simulink model "nms_model"  (Simulink 7.5)
settings: Solver=ode15s  StartTime=0.0  StopTime=60  FixedStep=1e-3  MaxStep=ts_max  RelTol=1e-3  AbsTol=1e-4
InitFcn:
  | nms_model_MechInit
  | nms_model_ControlInit
values from neighbouring files (symbols this model uses):
  c = 0.05    [muscleParams.m]    (also in nms_model_MechInit.m)
  c_jointstop = 0.3 / (pi/180)    (= 17.1887338539)    [muscleParams.m]    (also in nms_model_MechInit.m)
  D12_F = 0.16    [nms_model_MechInit.m]
  D12_S = L_S    (= 0.5)    [nms_model_MechInit.m]
  D12_T = L_T    (= 0.5)    [nms_model_MechInit.m]
  D13_F = 0.20    (= 0.2)    [nms_model_MechInit.m]
  D1G_F = 0.14    [nms_model_MechInit.m]
  D1G_HAT = 0.35    [nms_model_MechInit.m]
  D1G_S = 0.3    [nms_model_MechInit.m]
  D1G_T = 0.3    [nms_model_MechInit.m]
  DeltaThRef = 5e-3    (= 0.005)    [nms_model_MechInit.m]
  eref = 0.04    [muscleParams.m]    (also in nms_model_MechInit.m)
  FmaxGAS = 1500    [nms_model_MechInit.m]
  FmaxGLU = 1500    [nms_model_MechInit.m]
  FmaxHAM = 3000    [nms_model_MechInit.m]
  FmaxHFL = 2000    [nms_model_MechInit.m]
  FmaxSOL = 4000    [nms_model_MechInit.m]
  FmaxTA = 800    [nms_model_MechInit.m]
  FmaxVAS = 300    [muscleParams.m]    (also in nms_model_MechInit.m = 6000)
  GainDeltaTheta = 2 /100*180/pi    (= 1.14591559026)    [nms_model_ControlInit.m]
  GainGAS = 1.1/FmaxGAS    [nms_model_ControlInit.m]
  GainGLU = 0.5/FmaxGLU    [nms_model_ControlInit.m]
  GainHAM = 0.65/FmaxHAM    [nms_model_ControlInit.m]
  GainHAMHFL = 4    [nms_model_ControlInit.m]
  GainHFL = 0.5    [nms_model_ControlInit.m]
  GainKneOverExt = 2    [nms_model_ControlInit.m]
  GainSOL = 1.2/FmaxSOL    [nms_model_ControlInit.m]
  GainSOLTA = 0.4/FmaxSOL    [nms_model_ControlInit.m]
  GainTA = 1.1    [nms_model_ControlInit.m]
  GainVAS = 1.2/FmaxVAS    [nms_model_ControlInit.m]
  In_F = 0.005    [nms_model_MechInit.m]
  In_HAT = 3    [nms_model_MechInit.m]
  In_S = 0.05    [nms_model_MechInit.m]
  In_T = 0.15    [nms_model_MechInit.m]
  K = 5    [muscleParams.m]    (also in nms_model_MechInit.m)
  k_gx = (2*(m_F+m_S+m_T)+m_HAT)*g/0.1    (= 7848)    [nms_model_MechInit.m]
  k_gy = (2*(m_F+m_S+m_T)+m_HAT)*g/0.01    (= 78480)    [nms_model_MechInit.m]
  k_pressure = m_HAT * 9.81 / DeltaThRef    (= 104967)    [nms_model_MechInit.m]
  K_swing = 0.25    [nms_model_ControlInit.m]
  KneePh23Offset = 170*pi/180    (= 2.96705972839)    [nms_model_ControlInit.m]
  LceOffsetHAM = 0.85    [nms_model_ControlInit.m]
  LceOffsetHFL = 0.65    [nms_model_ControlInit.m]
  LceOffsetTA = 1-0.5*w    [nms_model_ControlInit.m]
  LongDelay = 0.020    (= 0.02)    [nms_model_ControlInit.m]
  loptGAS = 0.05    [nms_model_MechInit.m]
  loptGLU = 0.11    [nms_model_MechInit.m]
  loptHAM = 0.10    (= 0.1)    [nms_model_MechInit.m]
  loptHFL = 0.11    [nms_model_MechInit.m]
  loptSOL = 0.04    [nms_model_MechInit.m]
  loptTA = 0.06    [nms_model_MechInit.m]
  loptVAS = 0.13    [muscleParams.m]    (also in nms_model_MechInit.m = 0.08)
  lslackGAS = 0.40    (= 0.4)    [nms_model_MechInit.m]
  lslackGLU = 0.13    [nms_model_MechInit.m]
  lslackHAM = 0.31    [nms_model_MechInit.m]
  lslackHFL = 0.10    (= 0.1)    [nms_model_MechInit.m]
  lslackSOL = 0.26    [nms_model_MechInit.m]
  lslackTA = 0.24    [nms_model_MechInit.m]
  lslackVAS = 0.23    [muscleParams.m]    (also in nms_model_MechInit.m)
  m_F = 1.25    [nms_model_MechInit.m]
  m_HAT = 53.5    [nms_model_MechInit.m]
  m_S = 3.5    [nms_model_MechInit.m]
  m_T = 8.5    [nms_model_MechInit.m]
  MidDelay = 0.010    (= 0.01)    [nms_model_ControlInit.m]
  mu_slide = 0.8    [nms_model_MechInit.m]
  mu_stick = 0.9    [nms_model_MechInit.m]
  N = 1.5    [muscleParams.m]    (also in nms_model_MechInit.m)
  phi12_LowLimit = 70*pi/180    (= 1.2217304764)    [nms_model_MechInit.m]
  phi12_UpLimit = 180*pi/180    (= 3.14159265359)    [muscleParams.m]    (also in nms_model_MechInit.m = 2.26892802759)
  phi23_UpLimit = 159*pi/180    (= 2.77507351067)    [muscleParams.m]    (also in nms_model_MechInit.m = 3.05432619099)
  phi34_UpLimit = 230*pi/180    (= 4.01425727959)    [nms_model_MechInit.m]
  phimaxGASa = 110*pi/180    (= 1.91986217719)    [nms_model_MechInit.m]
  phimaxGASk = 140*pi/180    (= 2.44346095279)    [nms_model_MechInit.m]
  phimaxHAMk = 180*pi/180    (= 3.14159265359)    [nms_model_MechInit.m]
  phimaxSOL = 110*pi/180    (= 1.91986217719)    [nms_model_MechInit.m]
  phimaxTA = 80*pi/180    (= 1.3962634016)    [nms_model_MechInit.m]
  phimaxVAS = 90*pi/180    (= 1.57079632679)    [muscleParams.m]    (also in nms_model_MechInit.m = 2.87979326579)
  phirefGASa = 80*pi/180    (= 1.3962634016)    [nms_model_MechInit.m]
  phirefGASk = 165*pi/180    (= 2.87979326579)    [nms_model_MechInit.m]
  phirefGLU = 150*pi/180    (= 2.61799387799)    [nms_model_MechInit.m]
  phirefHAMh = 155*pi/180    (= 2.70526034059)    [nms_model_MechInit.m]
  phirefHAMk = 180*pi/180    (= 3.14159265359)    [nms_model_MechInit.m]
  phirefHFL = 180*pi/180    (= 3.14159265359)    [nms_model_MechInit.m]
  phirefSOL = 80*pi/180    (= 1.3962634016)    [nms_model_MechInit.m]
  phirefTA = 110*pi/180    (= 1.91986217719)    [nms_model_MechInit.m]
  phirefVAS = 60*pi/180    (= 1.0471975512)    [muscleParams.m]    (also in nms_model_MechInit.m = 2.18166156499)
  PosGainGG = 1/(30*pi/180)    (= 1.9098593171)    [nms_model_ControlInit.m]
  PreStimGAS = 0.01    [nms_model_ControlInit.m]
  PreStimGG = 0.05    [nms_model_ControlInit.m]
  PreStimGLU = 0.01    [nms_model_ControlInit.m]
  PreStimHAM = 0.01    [nms_model_ControlInit.m]
  PreStimHFL = 0.01    [nms_model_ControlInit.m]
  PreStimSOL = 0.01    [nms_model_ControlInit.m]
  PreStimTA = 0.01    [nms_model_ControlInit.m]
  PreStimVAS = 0.08    [nms_model_ControlInit.m]
  rGASa = 0.05    [nms_model_MechInit.m]
  rGASk = 0.05    [nms_model_MechInit.m]
  rGLU = 0.10    (= 0.1)    [nms_model_MechInit.m]
  rHAMh = 0.08    [nms_model_MechInit.m]
  rHAMk = 0.05    [nms_model_MechInit.m]
  rHFL = 0.10    (= 0.1)    [nms_model_MechInit.m]
  rhoGASa = 0.7    [nms_model_MechInit.m]
  rhoGASk = 0.7    [nms_model_MechInit.m]
  rhoGLU = 0.5    [nms_model_MechInit.m]
  rhoHAMh = 0.7    [nms_model_MechInit.m]
  rhoHAMk = 0.7    [nms_model_MechInit.m]
  rhoHFL = 0.5    [nms_model_MechInit.m]
  rhoSOL = 0.5    [nms_model_MechInit.m]
  rhoTA = 0.7    [nms_model_MechInit.m]
  rhoVAS = 3    [muscleParams.m]    (also in nms_model_MechInit.m = 0.7)
  rSOL = 0.05    [nms_model_MechInit.m]
  rTA = 0.04    [nms_model_MechInit.m]
  rVAS = 0.03    [muscleParams.m]    (also in nms_model_MechInit.m = 0.06)
  s = orProblemSendCommand(['LoadIKFastSolver robot Translation3D'],probid)    [init.m]
  ShortDelay = 0.005    [nms_model_ControlInit.m]
  SpeedGainGG = 0.2    [nms_model_ControlInit.m]
  tau = 0.01    [muscleParams.m]    (also in nms_model_MechInit.m)
  Theta0 = 6*pi/180    (= 0.10471975512)    [nms_model_ControlInit.m]
  ThPos = 4/5    (= 0.8)    [nms_model_MechInit.m]
  v_gx_max = 0.03    [nms_model_MechInit.m]
  v_gy_max = 0.03    [nms_model_MechInit.m]
  ... (+11 more)
undefined symbols (not defined in the file or in its folder): sgn
libraries: mblibv1 x60, simulink x22, simulink_extras x20
(part 8 of 9)

== system nms_model/Muscle Actuation Layer/R HAM/BE force-length relation ==
  note: Buffer Elasticity BE
  lce [lopt] : Inport  OutDataType=sfix(16)  OutScaling=2^0
  Constant1 : Constant  Value=1-w  OutDataType=sfix(16)  OutScaling=2^0
  Math Function : Math  Operator=square  OutDataType=sfix(16)  OutScaling=2^0  SaturateOnIntegerOverflow=on
  Mux1 : Mux  Inputs=2
  Sum4 : Sum  Inputs=|+-  OutDataType=sfix(16)  OutScaling=2^0  SaturateOnIntegerOverflow=on  InputSameDT=on  OutDataTypeStr=Inherit: Same as first input
  force above slack length : Fcn  Expr=u(2)*(u(1)<0)
  reference strain [lslack] : Constant  Value=w/2  OutDataType=sfix(16)  OutScaling=2^0
  relative strain : Product  Inputs=*/  OutDataType=sfix(16)  OutScaling=2^-10
  fbe [Fmax] : Outport  OutDataType=sfix(16)  OutScaling=2^0
  wires:
  lce [lopt]/1 -> Sum4/1
  Mux1/1 -> force above slack length/1
  force above slack length/1 -> fbe [Fmax]/1
  Math Function/1 -> Mux1/2
  relative strain/1 -> Math Function/1
  reference strain [lslack]/1 -> relative strain/2
  Sum4/1 -> relative strain/1, Mux1/1
  Constant1/1 -> Sum4/2

== system nms_model/Muscle Actuation Layer/R HAM/CE force-length relation ==
  note: CE Force-Length Relationship
  lce [lopt] : Inport  OutDataType=sfix(16)  OutScaling=2^0
  Abs : Abs
  Constant1 : Constant  OutDataType=sfix(16)  OutScaling=2^0
  Constant2 : Constant  Value=3  OutDataType=sfix(16)  OutScaling=2^0
  Gain : Gain  Gain=log(c)  ParameterDataType=sfix(16)  ParameterScaling=2^0  OutDataType=sfix(16)  OutScaling=2^0
  Math Function : Math  OutDataType=sfix(16)  OutScaling=2^0  SaturateOnIntegerOverflow=on
  Math Function1 : Math  Operator=pow  OutDataType=sfix(16)  OutScaling=2^0  SaturateOnIntegerOverflow=on
  Sum4 : Sum  Inputs=|+-  OutDataType=sfix(16)  OutScaling=2^0  SaturateOnIntegerOverflow=on  InputSameDT=on  OutDataTypeStr=Inherit: Same as first input
  normalized position : Product  Inputs=*/  OutDataType=sfix(16)  OutScaling=2^-10
  relative width : Constant  Value=w  OutDataType=sfix(16)  OutScaling=2^0
  fce [Fmax] : Outport  OutDataType=sfix(16)  OutScaling=2^0
  wires:
  lce [lopt]/1 -> Sum4/1
  relative width/1 -> normalized position/2
  Constant1/1 -> Sum4/2
  Sum4/1 -> Abs/1
  Abs/1 -> normalized position/1
  normalized position/1 -> Math Function1/1
  Constant2/1 -> Math Function1/2
  Math Function1/1 -> Gain/1
  Gain/1 -> Math Function/1
  Math Function/1 -> fce [Fmax]/1

== system nms_model/Muscle Actuation Layer/R HAM/CE inverse  force-velocity relation ==
  note: CE Inverse Force-Velocity Relationship
  Fv[Fmax] : Inport  OutDataType=sfix(16)  OutScaling=2^0
  1 : Product  Inputs=/*  OutDataType=sfix(16)  OutScaling=2^-10
  Constant{1,3..4,8} (4 alike) : Constant  OutDataType=sfix(16)  OutScaling=2^0
  Constant2 : Constant  Value=N  OutDataType=sfix(16)  OutScaling=2^0
  Constant5 : Constant  Value=N  OutDataType=sfix(16)  OutScaling=2^0
  Curvature : Gain  Gain=K  ParameterDataType=sfix(16)  ParameterScaling=2^0  OutDataType=sfix(16)  OutScaling=2^0  SaturateOnIntegerOverflow=on  OutDataTypeStr=Inherit: Same as input  ParamDataTypeStr=Inherit: Same as input
  Curvature1 : Gain  Gain=7.56*K  ParameterDataType=sfix(16)  ParameterScaling=2^0  OutDataType=sfix(16)  OutScaling=2^0  SaturateOnIntegerOverflow=on  OutDataTypeStr=Inherit: Same as input  ParamDataTypeStr=Inherit: Same as input
  Mux : Mux  Inputs=2
  Mux1 : Mux  Inputs=3
  Mux2 : Mux  Inputs=3
  Slope : Gain  Gain=1e-2  ParameterDataType=sfix(16)  ParameterScaling=2^0  OutDataType=sfix(16)  OutScaling=2^0  SaturateOnIntegerOverflow=on  OutDataTypeStr=Inherit: Same as input  ParamDataTypeStr=Inherit: Same as input
  Sum1 : Sum  Inputs=|++  OutDataType=sfix(16)  OutScaling=2^0  SaturateOnIntegerOverflow=on  InputSameDT=on  OutDataTypeStr=Inherit: Same as first input
  Sum2 : Sum  OutDataType=sfix(16)  OutScaling=2^0  SaturateOnIntegerOverflow=on  InputSameDT=on  OutDataTypeStr=Inherit: Same as first input
  Sum3 : Sum  Inputs=++|  OutDataType=sfix(16)  OutScaling=2^0  SaturateOnIntegerOverflow=on  InputSameDT=on  OutDataTypeStr=Inherit: Same as first input
  Sum4 : Sum  Inputs=|+-  OutDataType=sfix(16)  OutScaling=2^0  SaturateOnIntegerOverflow=on  InputSameDT=on  OutDataTypeStr=Inherit: Same as first input
  Sum5 : Sum  Inputs=|-+  OutDataType=sfix(16)  OutScaling=2^0  SaturateOnIntegerOverflow=on  InputSameDT=on  OutDataTypeStr=Inherit: Same as first input
  Sum6 : Sum  Inputs=-+|  OutDataType=sfix(16)  OutScaling=2^0  SaturateOnIntegerOverflow=on  InputSameDT=on  OutDataTypeStr=Inherit: Same as first input
  Sum7 : Sum  Inputs=|++  OutDataType=sfix(16)  OutScaling=2^0  SaturateOnIntegerOverflow=on  InputSameDT=on  OutDataTypeStr=Inherit: Same as first input
  Sum8 : Sum  Inputs=+-|  OutDataType=sfix(16)  OutScaling=2^0  SaturateOnIntegerOverflow=on  InputSameDT=on  OutDataTypeStr=Inherit: Same as first input
  Sum9 : Sum  OutDataType=sfix(16)  OutScaling=2^0  SaturateOnIntegerOverflow=on  InputSameDT=on  OutDataTypeStr=Inherit: Same as first input
  concentric branch : Fcn  Expr=u(1) * (u(2)<=1)
  excentric branch : Fcn  Expr=u(2) * (u(1)>1)*(u(1)<=u(3))
  excentric overshoot : Fcn  Expr=u(3) * (u(2)>u(1))
  v_concentric : Product  Inputs=*/  OutDataType=sfix(16)  OutScaling=2^-10
  v_excentric <N : Product  Inputs=*/  OutDataType=sfix(16)  OutScaling=2^-10
  v[vmax] : Outport  OutDataType=sfix(16)  OutScaling=2^0
  wires:
  Curvature/1 -> Sum3/2
  Constant1/1 -> Sum4/2, Sum3/1
  Sum4/1 -> v_concentric/1
  Sum3/1 -> v_concentric/2
  1/1 -> Sum7/1, Curvature1/1
  Constant4/1 -> Sum7/2, Sum8/1
  Curvature1/1 -> Sum8/2
  Sum8/1 -> v_excentric <N/2
  Sum7/1 -> v_excentric <N/1
  v_concentric/1 -> Mux/1
  Fv[Fmax]/1 -> Sum4/1, Curvature/1, Sum6/2, Mux/2, Mux1/1, Mux2/2
  Sum9/1 -> v[vmax]/1
  Sum2/1 -> Sum9/2
  excentric overshoot/1 -> Sum2/2
  Slope/1 -> Sum1/1
  Constant8/1 -> Sum1/2
  Sum6/1 -> 1/2, Slope/1
  Constant2/1 -> Sum6/1, Sum5/2
  Sum5/1 -> 1/1
  Constant3/1 -> Sum5/1
  Mux/1 -> concentric branch/1
  Mux1/1 -> excentric branch/1
  v_excentric <N/1 -> Mux1/2
  Mux2/1 -> excentric overshoot/1
  concentric branch/1 -> Sum9/1
  excentric branch/1 -> Sum2/1
  Constant5/1 -> Mux1/3, Mux2/1
  Sum1/1 -> Mux2/3

== system nms_model/Muscle Actuation Layer/R HAM/PE force-length relation ==
  note: Parallel Elasticity PE
  lce [lopt] : Inport  OutDataType=sfix(16)  OutScaling=2^0
  Constant3 : Constant  OutDataType=sfix(16)  OutScaling=2^0
  Math Function2 : Math  Operator=square  OutDataType=sfix(16)  OutScaling=2^0  SaturateOnIntegerOverflow=on
  Mux : Mux  Inputs=2
  Sum1 : Sum  Inputs=|+-  OutDataType=sfix(16)  OutScaling=2^0  SaturateOnIntegerOverflow=on  InputSameDT=on  OutDataTypeStr=Inherit: Same as first input
  force above slack length : Fcn  Expr=u(2) * (u(1)>1)
  reference strain [lopt] : Constant  Value=w  OutDataType=sfix(16)  OutScaling=2^0
  relative strain : Product  Inputs=*/  OutDataType=sfix(16)  OutScaling=2^-10
  fpe [Fmax] : Outport  OutDataType=sfix(16)  OutScaling=2^0
  wires:
  Mux/1 -> force above slack length/1
  lce [lopt]/1 -> Mux/1, Sum1/1
  Constant3/1 -> Sum1/2
  Sum1/1 -> relative strain/1
  reference strain [lopt]/1 -> relative strain/2
  relative strain/1 -> Math Function2/1
  Math Function2/1 -> Mux/2
  force above slack length/1 -> fpe [Fmax]/1

== system nms_model/Muscle Actuation Layer/R HAM/SE force-length relation ==
  note: SE Force-Length Relationship
  lse [lslack] : Inport  OutDataType=sfix(16)  OutScaling=2^0
  Constant1 : Constant  OutDataType=sfix(16)  OutScaling=2^0
  Math Function : Math  Operator=square  OutDataType=sfix(16)  OutScaling=2^0  SaturateOnIntegerOverflow=on
  Mux : Mux  Inputs=2
  Sum4 : Sum  Inputs=|+-  OutDataType=sfix(16)  OutScaling=2^0  SaturateOnIntegerOverflow=on  InputSameDT=on  OutDataTypeStr=Inherit: Same as first input
  force above slack length : Fcn  Expr=u(2)*(u(1)>1)
  reference strain [lslack] : Constant  Value=eref  OutDataType=sfix(16)  OutScaling=2^0
  relative strain : Product  Inputs=*/  OutDataType=sfix(16)  OutScaling=2^-10
  fse [Fmax] : Outport  OutDataType=sfix(16)  OutScaling=2^0
  wires:
  Mux/1 -> force above slack length/1
  force above slack length/1 -> fse [Fmax]/1
  Math Function/1 -> Mux/2
  lse [lslack]/1 -> Mux/1, Sum4/1
  relative strain/1 -> Math Function/1
  reference strain [lslack]/1 -> relative strain/2
  Sum4/1 -> relative strain/1
  Constant1/1 -> Sum4/2

== system nms_model/Muscle Actuation Layer/R HFL/BE force-length relation ==
  note: Buffer Elasticity BE
  lce [lopt] : Inport  OutDataType=sfix(16)  OutScaling=2^0
  Constant1 : Constant  Value=1-w  OutDataType=sfix(16)  OutScaling=2^0
  Math Function : Math  Operator=square  OutDataType=sfix(16)  OutScaling=2^0  SaturateOnIntegerOverflow=on
  Mux1 : Mux  Inputs=2
  Sum4 : Sum  Inputs=|+-  OutDataType=sfix(16)  OutScaling=2^0  SaturateOnIntegerOverflow=on  InputSameDT=on  OutDataTypeStr=Inherit: Same as first input
  force above slack length : Fcn  Expr=u(2)*(u(1)<0)
  reference strain [lslack] : Constant  Value=w/2  OutDataType=sfix(16)  OutScaling=2^0
  relative strain : Product  Inputs=*/  OutDataType=sfix(16)  OutScaling=2^-10
  fbe [Fmax] : Outport  OutDataType=sfix(16)  OutScaling=2^0
  wires:
  lce [lopt]/1 -> Sum4/1
  Mux1/1 -> force above slack length/1
  force above slack length/1 -> fbe [Fmax]/1
  Math Function/1 -> Mux1/2
  relative strain/1 -> Math Function/1
  reference strain [lslack]/1 -> relative strain/2
  Sum4/1 -> relative strain/1, Mux1/1
  Constant1/1 -> Sum4/2

== system nms_model/Muscle Actuation Layer/R HFL/CE force-length relation ==
  note: CE Force-Length Relationship
  lce [lopt] : Inport  OutDataType=sfix(16)  OutScaling=2^0
  Abs : Abs
  Constant1 : Constant  OutDataType=sfix(16)  OutScaling=2^0
  Constant2 : Constant  Value=3  OutDataType=sfix(16)  OutScaling=2^0
  Gain : Gain  Gain=log(c)  ParameterDataType=sfix(16)  ParameterScaling=2^0  OutDataType=sfix(16)  OutScaling=2^0
  Math Function : Math  OutDataType=sfix(16)  OutScaling=2^0  SaturateOnIntegerOverflow=on
  Math Function1 : Math  Operator=pow  OutDataType=sfix(16)  OutScaling=2^0  SaturateOnIntegerOverflow=on
  Sum4 : Sum  Inputs=|+-  OutDataType=sfix(16)  OutScaling=2^0  SaturateOnIntegerOverflow=on  InputSameDT=on  OutDataTypeStr=Inherit: Same as first input
  normalized position : Product  Inputs=*/  OutDataType=sfix(16)  OutScaling=2^-10
  relative width : Constant  Value=w  OutDataType=sfix(16)  OutScaling=2^0
  fce [Fmax] : Outport  OutDataType=sfix(16)  OutScaling=2^0
  wires:
  lce [lopt]/1 -> Sum4/1
  relative width/1 -> normalized position/2
  Constant1/1 -> Sum4/2
  Sum4/1 -> Abs/1
  Abs/1 -> normalized position/1
  normalized position/1 -> Math Function1/1
  Constant2/1 -> Math Function1/2
  Math Function1/1 -> Gain/1
  Gain/1 -> Math Function/1
  Math Function/1 -> fce [Fmax]/1

== system nms_model/Muscle Actuation Layer/R HFL/CE inverse  force-velocity relation ==
  note: CE Inverse Force-Velocity Relationship
  Fv[Fmax] : Inport  OutDataType=sfix(16)  OutScaling=2^0
  1 : Product  Inputs=/*  OutDataType=sfix(16)  OutScaling=2^-10
  Constant{1,3..4,8} (4 alike) : Constant  OutDataType=sfix(16)  OutScaling=2^0
  Constant2 : Constant  Value=N  OutDataType=sfix(16)  OutScaling=2^0
  Constant5 : Constant  Value=N  OutDataType=sfix(16)  OutScaling=2^0
  Curvature : Gain  Gain=K  ParameterDataType=sfix(16)  ParameterScaling=2^0  OutDataType=sfix(16)  OutScaling=2^0  SaturateOnIntegerOverflow=on  OutDataTypeStr=Inherit: Same as input  ParamDataTypeStr=Inherit: Same as input
  Curvature1 : Gain  Gain=7.56*K  ParameterDataType=sfix(16)  ParameterScaling=2^0  OutDataType=sfix(16)  OutScaling=2^0  SaturateOnIntegerOverflow=on  OutDataTypeStr=Inherit: Same as input  ParamDataTypeStr=Inherit: Same as input
  Mux : Mux  Inputs=2
  Mux1 : Mux  Inputs=3
  Mux2 : Mux  Inputs=3
  Slope : Gain  Gain=1e-2  ParameterDataType=sfix(16)  ParameterScaling=2^0  OutDataType=sfix(16)  OutScaling=2^0  SaturateOnIntegerOverflow=on  OutDataTypeStr=Inherit: Same as input  ParamDataTypeStr=Inherit: Same as input
  Sum1 : Sum  Inputs=|++  OutDataType=sfix(16)  OutScaling=2^0  SaturateOnIntegerOverflow=on  InputSameDT=on  OutDataTypeStr=Inherit: Same as first input
  Sum2 : Sum  OutDataType=sfix(16)  OutScaling=2^0  SaturateOnIntegerOverflow=on  InputSameDT=on  OutDataTypeStr=Inherit: Same as first input
  Sum3 : Sum  Inputs=++|  OutDataType=sfix(16)  OutScaling=2^0  SaturateOnIntegerOverflow=on  InputSameDT=on  OutDataTypeStr=Inherit: Same as first input
  Sum4 : Sum  Inputs=|+-  OutDataType=sfix(16)  OutScaling=2^0  SaturateOnIntegerOverflow=on  InputSameDT=on  OutDataTypeStr=Inherit: Same as first input
  Sum5 : Sum  Inputs=|-+  OutDataType=sfix(16)  OutScaling=2^0  SaturateOnIntegerOverflow=on  InputSameDT=on  OutDataTypeStr=Inherit: Same as first input
  Sum6 : Sum  Inputs=-+|  OutDataType=sfix(16)  OutScaling=2^0  SaturateOnIntegerOverflow=on  InputSameDT=on  OutDataTypeStr=Inherit: Same as first input
  Sum7 : Sum  Inputs=|++  OutDataType=sfix(16)  OutScaling=2^0  SaturateOnIntegerOverflow=on  InputSameDT=on  OutDataTypeStr=Inherit: Same as first input
  Sum8 : Sum  Inputs=+-|  OutDataType=sfix(16)  OutScaling=2^0  SaturateOnIntegerOverflow=on  InputSameDT=on  OutDataTypeStr=Inherit: Same as first input
  Sum9 : Sum  OutDataType=sfix(16)  OutScaling=2^0  SaturateOnIntegerOverflow=on  InputSameDT=on  OutDataTypeStr=Inherit: Same as first input
  concentric branch : Fcn  Expr=u(1) * (u(2)<=1)
  excentric branch : Fcn  Expr=u(2) * (u(1)>1)*(u(1)<=u(3))
  excentric overshoot : Fcn  Expr=u(3) * (u(2)>u(1))
  v_concentric : Product  Inputs=*/  OutDataType=sfix(16)  OutScaling=2^-10
  v_excentric <N : Product  Inputs=*/  OutDataType=sfix(16)  OutScaling=2^-10
  v[vmax] : Outport  OutDataType=sfix(16)  OutScaling=2^0
  wires:
  Curvature/1 -> Sum3/2
  Constant1/1 -> Sum4/2, Sum3/1
  Sum4/1 -> v_concentric/1
  Sum3/1 -> v_concentric/2
  1/1 -> Sum7/1, Curvature1/1
  Constant4/1 -> Sum7/2, Sum8/1
  Curvature1/1 -> Sum8/2
  Sum8/1 -> v_excentric <N/2
  Sum7/1 -> v_excentric <N/1
  v_concentric/1 -> Mux/1
  Fv[Fmax]/1 -> Sum4/1, Curvature/1, Sum6/2, Mux/2, Mux1/1, Mux2/2
  Sum9/1 -> v[vmax]/1
  Sum2/1 -> Sum9/2
  excentric overshoot/1 -> Sum2/2
  Slope/1 -> Sum1/1
  Constant8/1 -> Sum1/2
  Sum6/1 -> 1/2, Slope/1
  Constant2/1 -> Sum6/1, Sum5/2
  Sum5/1 -> 1/1
  Constant3/1 -> Sum5/1
  Mux/1 -> concentric branch/1
  Mux1/1 -> excentric branch/1
  v_excentric <N/1 -> Mux1/2
  Mux2/1 -> excentric overshoot/1
  concentric branch/1 -> Sum9/1
  excentric branch/1 -> Sum2/1
  Constant5/1 -> Mux1/3, Mux2/1
  Sum1/1 -> Mux2/3

== system nms_model/Muscle Actuation Layer/R HFL/PE force-length relation ==
  note: Parallel Elasticity PE
  lce [lopt] : Inport  OutDataType=sfix(16)  OutScaling=2^0
  Constant3 : Constant  OutDataType=sfix(16)  OutScaling=2^0
  Math Function2 : Math  Operator=square  OutDataType=sfix(16)  OutScaling=2^0  SaturateOnIntegerOverflow=on
  Mux : Mux  Inputs=2
  Sum1 : Sum  Inputs=|+-  OutDataType=sfix(16)  OutScaling=2^0  SaturateOnIntegerOverflow=on  InputSameDT=on  OutDataTypeStr=Inherit: Same as first input
  force above slack length : Fcn  Expr=u(2) * (u(1)>1)
  reference strain [lopt] : Constant  Value=w  OutDataType=sfix(16)  OutScaling=2^0
  relative strain : Product  Inputs=*/  OutDataType=sfix(16)  OutScaling=2^-10
  fpe [Fmax] : Outport  OutDataType=sfix(16)  OutScaling=2^0
  wires:
  Mux/1 -> force above slack length/1
  lce [lopt]/1 -> Mux/1, Sum1/1
  Constant3/1 -> Sum1/2
  Sum1/1 -> relative strain/1
  reference strain [lopt]/1 -> relative strain/2
  relative strain/1 -> Math Function2/1
  Math Function2/1 -> Mux/2
  force above slack length/1 -> fpe [Fmax]/1

== system nms_model/Muscle Actuation Layer/R HFL/SE force-length relation ==
  note: SE Force-Length Relationship
  lse [lslack] : Inport  OutDataType=sfix(16)  OutScaling=2^0
  Constant1 : Constant  OutDataType=sfix(16)  OutScaling=2^0
  Math Function : Math  Operator=square  OutDataType=sfix(16)  OutScaling=2^0  SaturateOnIntegerOverflow=on
  Mux : Mux  Inputs=2
  Sum4 : Sum  Inputs=|+-  OutDataType=sfix(16)  OutScaling=2^0  SaturateOnIntegerOverflow=on  InputSameDT=on  OutDataTypeStr=Inherit: Same as first input
  force above slack length : Fcn  Expr=u(2)*(u(1)>1)
  reference strain [lslack] : Constant  Value=eref  OutDataType=sfix(16)  OutScaling=2^0
  relative strain : Product  Inputs=*/  OutDataType=sfix(16)  OutScaling=2^-10
  fse [Fmax] : Outport  OutDataType=sfix(16)  OutScaling=2^0
  wires:
  Mux/1 -> force above slack length/1
  force above slack length/1 -> fse [Fmax]/1
  Math Function/1 -> Mux/2
  lse [lslack]/1 -> Mux/1, Sum4/1
  relative strain/1 -> Math Function/1
  reference strain [lslack]/1 -> relative strain/2
  Sum4/1 -> relative strain/1
  Constant1/1 -> Sum4/2

== system nms_model/Muscle Actuation Layer/R SOL/BE force-length relation ==
  note: Buffer Elasticity BE
  lce [lopt] : Inport  OutDataType=sfix(16)  OutScaling=2^0
  Constant1 : Constant  Value=1-w  OutDataType=sfix(16)  OutScaling=2^0
  Math Function : Math  Operator=square  OutDataType=sfix(16)  OutScaling=2^0  SaturateOnIntegerOverflow=on
  Mux1 : Mux  Inputs=2
  Sum4 : Sum  Inputs=|+-  OutDataType=sfix(16)  OutScaling=2^0  SaturateOnIntegerOverflow=on  InputSameDT=on  OutDataTypeStr=Inherit: Same as first input
  force above slack length : Fcn  Expr=u(2)*(u(1)<0)
  reference strain [lslack] : Constant  Value=w/2  OutDataType=sfix(16)  OutScaling=2^0
  relative strain : Product  Inputs=*/  OutDataType=sfix(16)  OutScaling=2^-10
  fbe [Fmax] : Outport  OutDataType=sfix(16)  OutScaling=2^0
  wires:
  lce [lopt]/1 -> Sum4/1
  Mux1/1 -> force above slack length/1
  force above slack length/1 -> fbe [Fmax]/1
  Math Function/1 -> Mux1/2
  relative strain/1 -> Math Function/1
  reference strain [lslack]/1 -> relative strain/2
  Sum4/1 -> relative strain/1, Mux1/1
  Constant1/1 -> Sum4/2

== system nms_model/Muscle Actuation Layer/R SOL/CE force-length relation ==
  note: CE Force-Length Relationship
  lce [lopt] : Inport  OutDataType=sfix(16)  OutScaling=2^0
  Abs : Abs
  Constant1 : Constant  OutDataType=sfix(16)  OutScaling=2^0
  Constant2 : Constant  Value=3  OutDataType=sfix(16)  OutScaling=2^0
  Gain : Gain  Gain=log(c)  ParameterDataType=sfix(16)  ParameterScaling=2^0  OutDataType=sfix(16)  OutScaling=2^0
  Math Function : Math  OutDataType=sfix(16)  OutScaling=2^0  SaturateOnIntegerOverflow=on
  Math Function1 : Math  Operator=pow  OutDataType=sfix(16)  OutScaling=2^0  SaturateOnIntegerOverflow=on
  Sum4 : Sum  Inputs=|+-  OutDataType=sfix(16)  OutScaling=2^0  SaturateOnIntegerOverflow=on  InputSameDT=on  OutDataTypeStr=Inherit: Same as first input
  normalized position : Product  Inputs=*/  OutDataType=sfix(16)  OutScaling=2^-10
  relative width : Constant  Value=w  OutDataType=sfix(16)  OutScaling=2^0
  fce [Fmax] : Outport  OutDataType=sfix(16)  OutScaling=2^0
  wires:
  lce [lopt]/1 -> Sum4/1
  relative width/1 -> normalized position/2
  Constant1/1 -> Sum4/2
  Sum4/1 -> Abs/1
  Abs/1 -> normalized position/1
  normalized position/1 -> Math Function1/1
  Constant2/1 -> Math Function1/2
  Math Function1/1 -> Gain/1
  Gain/1 -> Math Function/1
  Math Function/1 -> fce [Fmax]/1

== system nms_model/Muscle Actuation Layer/R SOL/CE inverse  force-velocity relation ==
  note: CE Inverse Force-Velocity Relationship
  Fv[Fmax] : Inport  OutDataType=sfix(16)  OutScaling=2^0
  1 : Product  Inputs=/*  OutDataType=sfix(16)  OutScaling=2^-10
  Constant{1,3..4,8} (4 alike) : Constant  OutDataType=sfix(16)  OutScaling=2^0
  Constant2 : Constant  Value=N  OutDataType=sfix(16)  OutScaling=2^0
  Constant5 : Constant  Value=N  OutDataType=sfix(16)  OutScaling=2^0
  Curvature : Gain  Gain=K  ParameterDataType=sfix(16)  ParameterScaling=2^0  OutDataType=sfix(16)  OutScaling=2^0  SaturateOnIntegerOverflow=on  OutDataTypeStr=Inherit: Same as input  ParamDataTypeStr=Inherit: Same as input
  Curvature1 : Gain  Gain=7.56*K  ParameterDataType=sfix(16)  ParameterScaling=2^0  OutDataType=sfix(16)  OutScaling=2^0  SaturateOnIntegerOverflow=on  OutDataTypeStr=Inherit: Same as input  ParamDataTypeStr=Inherit: Same as input
  Mux : Mux  Inputs=2
  Mux1 : Mux  Inputs=3
  Mux2 : Mux  Inputs=3
  Slope : Gain  Gain=1e-2  ParameterDataType=sfix(16)  ParameterScaling=2^0  OutDataType=sfix(16)  OutScaling=2^0  SaturateOnIntegerOverflow=on  OutDataTypeStr=Inherit: Same as input  ParamDataTypeStr=Inherit: Same as input
  Sum1 : Sum  Inputs=|++  OutDataType=sfix(16)  OutScaling=2^0  SaturateOnIntegerOverflow=on  InputSameDT=on  OutDataTypeStr=Inherit: Same as first input
  Sum2 : Sum  OutDataType=sfix(16)  OutScaling=2^0  SaturateOnIntegerOverflow=on  InputSameDT=on  OutDataTypeStr=Inherit: Same as first input
  Sum3 : Sum  Inputs=++|  OutDataType=sfix(16)  OutScaling=2^0  SaturateOnIntegerOverflow=on  InputSameDT=on  OutDataTypeStr=Inherit: Same as first input
  Sum4 : Sum  Inputs=|+-  OutDataType=sfix(16)  OutScaling=2^0  SaturateOnIntegerOverflow=on  InputSameDT=on  OutDataTypeStr=Inherit: Same as first input
  Sum5 : Sum  Inputs=|-+  OutDataType=sfix(16)  OutScaling=2^0  SaturateOnIntegerOverflow=on  InputSameDT=on  OutDataTypeStr=Inherit: Same as first input
  Sum6 : Sum  Inputs=-+|  OutDataType=sfix(16)  OutScaling=2^0  SaturateOnIntegerOverflow=on  InputSameDT=on  OutDataTypeStr=Inherit: Same as first input
  Sum7 : Sum  Inputs=|++  OutDataType=sfix(16)  OutScaling=2^0  SaturateOnIntegerOverflow=on  InputSameDT=on  OutDataTypeStr=Inherit: Same as first input
  Sum8 : Sum  Inputs=+-|  OutDataType=sfix(16)  OutScaling=2^0  SaturateOnIntegerOverflow=on  InputSameDT=on  OutDataTypeStr=Inherit: Same as first input
  Sum9 : Sum  OutDataType=sfix(16)  OutScaling=2^0  SaturateOnIntegerOverflow=on  InputSameDT=on  OutDataTypeStr=Inherit: Same as first input
  concentric branch : Fcn  Expr=u(1) * (u(2)<=1)
  excentric branch : Fcn  Expr=u(2) * (u(1)>1)*(u(1)<=u(3))
  excentric overshoot : Fcn  Expr=u(3) * (u(2)>u(1))
  v_concentric : Product  Inputs=*/  OutDataType=sfix(16)  OutScaling=2^-10
  v_excentric <N : Product  Inputs=*/  OutDataType=sfix(16)  OutScaling=2^-10
  v[vmax] : Outport  OutDataType=sfix(16)  OutScaling=2^0
  wires:
  Curvature/1 -> Sum3/2
  Constant1/1 -> Sum4/2, Sum3/1
  Sum4/1 -> v_concentric/1
  Sum3/1 -> v_concentric/2
  1/1 -> Sum7/1, Curvature1/1
  Constant4/1 -> Sum7/2, Sum8/1
  Curvature1/1 -> Sum8/2
  Sum8/1 -> v_excentric <N/2
  Sum7/1 -> v_excentric <N/1
  v_concentric/1 -> Mux/1
  Fv[Fmax]/1 -> Sum4/1, Curvature/1, Sum6/2, Mux/2, Mux1/1, Mux2/2
  Sum9/1 -> v[vmax]/1
  Sum2/1 -> Sum9/2
  excentric overshoot/1 -> Sum2/2
  Slope/1 -> Sum1/1
  Constant8/1 -> Sum1/2
  Sum6/1 -> 1/2, Slope/1
  Constant2/1 -> Sum6/1, Sum5/2
  Sum5/1 -> 1/1
  Constant3/1 -> Sum5/1
  Mux/1 -> concentric branch/1
  Mux1/1 -> excentric branch/1
  v_excentric <N/1 -> Mux1/2
  Mux2/1 -> excentric overshoot/1
  concentric branch/1 -> Sum9/1
  excentric branch/1 -> Sum2/1
  Constant5/1 -> Mux1/3, Mux2/1
  Sum1/1 -> Mux2/3

== system nms_model/Muscle Actuation Layer/R SOL/PE force-length relation ==
  note: Parallel Elasticity PE
  lce [lopt] : Inport  OutDataType=sfix(16)  OutScaling=2^0
  Constant3 : Constant  OutDataType=sfix(16)  OutScaling=2^0
  Math Function2 : Math  Operator=square  OutDataType=sfix(16)  OutScaling=2^0  SaturateOnIntegerOverflow=on
  Mux : Mux  Inputs=2
  Sum1 : Sum  Inputs=|+-  OutDataType=sfix(16)  OutScaling=2^0  SaturateOnIntegerOverflow=on  InputSameDT=on  OutDataTypeStr=Inherit: Same as first input
  force above slack length : Fcn  Expr=u(2) * (u(1)>1)
  reference strain [lopt] : Constant  Value=w  OutDataType=sfix(16)  OutScaling=2^0
  relative strain : Product  Inputs=*/  OutDataType=sfix(16)  OutScaling=2^-10
  fpe [Fmax] : Outport  OutDataType=sfix(16)  OutScaling=2^0
  wires:
  Mux/1 -> force above slack length/1
  lce [lopt]/1 -> Mux/1, Sum1/1
  Constant3/1 -> Sum1/2
  Sum1/1 -> relative strain/1
  reference strain [lopt]/1 -> relative strain/2
  relative strain/1 -> Math Function2/1
  Math Function2/1 -> Mux/2
  force above slack length/1 -> fpe [Fmax]/1

== system nms_model/Muscle Actuation Layer/R SOL/SE force-length relation ==
  note: SE Force-Length Relationship
  lse [lslack] : Inport  OutDataType=sfix(16)  OutScaling=2^0
  Constant1 : Constant  OutDataType=sfix(16)  OutScaling=2^0
  Math Function : Math  Operator=square  OutDataType=sfix(16)  OutScaling=2^0  SaturateOnIntegerOverflow=on
  Mux : Mux  Inputs=2
  Sum4 : Sum  Inputs=|+-  OutDataType=sfix(16)  OutScaling=2^0  SaturateOnIntegerOverflow=on  InputSameDT=on  OutDataTypeStr=Inherit: Same as first input
  force above slack length : Fcn  Expr=u(2)*(u(1)>1)
  reference strain [lslack] : Constant  Value=eref  OutDataType=sfix(16)  OutScaling=2^0
  relative strain : Product  Inputs=*/  OutDataType=sfix(16)  OutScaling=2^-10
  fse [Fmax] : Outport  OutDataType=sfix(16)  OutScaling=2^0
  wires:
  Mux/1 -> force above slack length/1
  force above slack length/1 -> fse [Fmax]/1
  Math Function/1 -> Mux/2
  lse [lslack]/1 -> Mux/1, Sum4/1
  relative strain/1 -> Math Function/1
  reference strain [lslack]/1 -> relative strain/2
  Sum4/1 -> relative strain/1
  Constant1/1 -> Sum4/2

== system nms_model/Muscle Actuation Layer/R TA/BE force-length relation ==
  note: Buffer Elasticity BE
  lce [lopt] : Inport  OutDataType=sfix(16)  OutScaling=2^0
  Constant1 : Constant  Value=1-w  OutDataType=sfix(16)  OutScaling=2^0
  Math Function : Math  Operator=square  OutDataType=sfix(16)  OutScaling=2^0  SaturateOnIntegerOverflow=on
  Mux1 : Mux  Inputs=2
  Sum4 : Sum  Inputs=|+-  OutDataType=sfix(16)  OutScaling=2^0  SaturateOnIntegerOverflow=on  InputSameDT=on  OutDataTypeStr=Inherit: Same as first input
  force above slack length : Fcn  Expr=u(2)*(u(1)<0)
  reference strain [lslack] : Constant  Value=w/2  OutDataType=sfix(16)  OutScaling=2^0
  relative strain : Product  Inputs=*/  OutDataType=sfix(16)  OutScaling=2^-10
  fbe [Fmax] : Outport  OutDataType=sfix(16)  OutScaling=2^0
  wires:
  lce [lopt]/1 -> Sum4/1
  Mux1/1 -> force above slack length/1
  force above slack length/1 -> fbe [Fmax]/1
  Math Function/1 -> Mux1/2
  relative strain/1 -> Math Function/1
  reference strain [lslack]/1 -> relative strain/2
  Sum4/1 -> relative strain/1, Mux1/1
  Constant1/1 -> Sum4/2

== system nms_model/Muscle Actuation Layer/R TA/CE force-length relation ==
  note: CE Force-Length Relationship
  lce [lopt] : Inport  OutDataType=sfix(16)  OutScaling=2^0
  Abs : Abs
  Constant1 : Constant  OutDataType=sfix(16)  OutScaling=2^0
  Constant2 : Constant  Value=3  OutDataType=sfix(16)  OutScaling=2^0
  Gain : Gain  Gain=log(c)  ParameterDataType=sfix(16)  ParameterScaling=2^0  OutDataType=sfix(16)  OutScaling=2^0
  Math Function : Math  OutDataType=sfix(16)  OutScaling=2^0  SaturateOnIntegerOverflow=on
  Math Function1 : Math  Operator=pow  OutDataType=sfix(16)  OutScaling=2^0  SaturateOnIntegerOverflow=on
  Sum4 : Sum  Inputs=|+-  OutDataType=sfix(16)  OutScaling=2^0  SaturateOnIntegerOverflow=on  InputSameDT=on  OutDataTypeStr=Inherit: Same as first input
  normalized position : Product  Inputs=*/  OutDataType=sfix(16)  OutScaling=2^-10
  relative width : Constant  Value=w  OutDataType=sfix(16)  OutScaling=2^0
  fce [Fmax] : Outport  OutDataType=sfix(16)  OutScaling=2^0
  wires:
  Math Function/1 -> fce [Fmax]/1
  Gain/1 -> Math Function/1
  Math Function1/1 -> Gain/1
  Constant2/1 -> Math Function1/2
  normalized position/1 -> Math Function1/1
  Abs/1 -> normalized position/1
  Sum4/1 -> Abs/1
  Constant1/1 -> Sum4/2
  relative width/1 -> normalized position/2
  lce [lopt]/1 -> Sum4/1

== system nms_model/Muscle Actuation Layer/R TA/CE inverse  force-velocity relation ==
  note: CE Inverse Force-Velocity Relationship
  Fv[Fmax] : Inport  OutDataType=sfix(16)  OutScaling=2^0
  1 : Product  Inputs=/*  OutDataType=sfix(16)  OutScaling=2^-10
  Constant{1,3..4,8} (4 alike) : Constant  OutDataType=sfix(16)  OutScaling=2^0
  Constant2 : Constant  Value=N  OutDataType=sfix(16)  OutScaling=2^0
  Constant5 : Constant  Value=N  OutDataType=sfix(16)  OutScaling=2^0
  Curvature : Gain  Gain=K  ParameterDataType=sfix(16)  ParameterScaling=2^0  OutDataType=sfix(16)  OutScaling=2^0  SaturateOnIntegerOverflow=on  OutDataTypeStr=Inherit: Same as input  ParamDataTypeStr=Inherit: Same as input
  Curvature1 : Gain  Gain=7.56*K  ParameterDataType=sfix(16)  ParameterScaling=2^0  OutDataType=sfix(16)  OutScaling=2^0  SaturateOnIntegerOverflow=on  OutDataTypeStr=Inherit: Same as input  ParamDataTypeStr=Inherit: Same as input
  Mux : Mux  Inputs=2
  Mux1 : Mux  Inputs=3
  Mux2 : Mux  Inputs=3
  Slope : Gain  Gain=1e-2  ParameterDataType=sfix(16)  ParameterScaling=2^0  OutDataType=sfix(16)  OutScaling=2^0  SaturateOnIntegerOverflow=on  OutDataTypeStr=Inherit: Same as input  ParamDataTypeStr=Inherit: Same as input
  Sum1 : Sum  Inputs=|++  OutDataType=sfix(16)  OutScaling=2^0  SaturateOnIntegerOverflow=on  InputSameDT=on  OutDataTypeStr=Inherit: Same as first input
  Sum2 : Sum  OutDataType=sfix(16)  OutScaling=2^0  SaturateOnIntegerOverflow=on  InputSameDT=on  OutDataTypeStr=Inherit: Same as first input
  Sum3 : Sum  Inputs=++|  OutDataType=sfix(16)  OutScaling=2^0  SaturateOnIntegerOverflow=on  InputSameDT=on  OutDataTypeStr=Inherit: Same as first input
  Sum4 : Sum  Inputs=|+-  OutDataType=sfix(16)  OutScaling=2^0  SaturateOnIntegerOverflow=on  InputSameDT=on  OutDataTypeStr=Inherit: Same as first input
  Sum5 : Sum  Inputs=|-+  OutDataType=sfix(16)  OutScaling=2^0  SaturateOnIntegerOverflow=on  InputSameDT=on  OutDataTypeStr=Inherit: Same as first input
  Sum6 : Sum  Inputs=-+|  OutDataType=sfix(16)  OutScaling=2^0  SaturateOnIntegerOverflow=on  InputSameDT=on  OutDataTypeStr=Inherit: Same as first input
  Sum7 : Sum  Inputs=|++  OutDataType=sfix(16)  OutScaling=2^0  SaturateOnIntegerOverflow=on  InputSameDT=on  OutDataTypeStr=Inherit: Same as first input
  Sum8 : Sum  Inputs=+-|  OutDataType=sfix(16)  OutScaling=2^0  SaturateOnIntegerOverflow=on  InputSameDT=on  OutDataTypeStr=Inherit: Same as first input
  Sum9 : Sum  OutDataType=sfix(16)  OutScaling=2^0  SaturateOnIntegerOverflow=on  InputSameDT=on  OutDataTypeStr=Inherit: Same as first input
  concentric branch : Fcn  Expr=u(1) * (u(2)<=1)
  excentric branch : Fcn  Expr=u(2) * (u(1)>1)*(u(1)<=u(3))
  excentric overshoot : Fcn  Expr=u(3) * (u(2)>u(1))
  v_concentric : Product  Inputs=*/  OutDataType=sfix(16)  OutScaling=2^-10
  v_excentric <N : Product  Inputs=*/  OutDataType=sfix(16)  OutScaling=2^-10
  v[vmax] : Outport  OutDataType=sfix(16)  OutScaling=2^0
  wires:
  Sum1/1 -> Mux2/3
  Constant5/1 -> Mux2/1, Mux1/3
  excentric branch/1 -> Sum2/1
  concentric branch/1 -> Sum9/1
  Mux2/1 -> excentric overshoot/1
  v_excentric <N/1 -> Mux1/2
  Mux1/1 -> excentric branch/1
  Mux/1 -> concentric branch/1
  Constant3/1 -> Sum5/1
  Sum5/1 -> 1/1
  Constant2/1 -> Sum5/2, Sum6/1
  Sum6/1 -> Slope/1, 1/2
  Constant8/1 -> Sum1/2
  Slope/1 -> Sum1/1
  excentric overshoot/1 -> Sum2/2
  Sum2/1 -> Sum9/2
  Sum9/1 -> v[vmax]/1
  Fv[Fmax]/1 -> Mux2/2, Mux1/1, Mux/2, Sum6/2, Curvature/1, Sum4/1
  v_concentric/1 -> Mux/1
  Sum7/1 -> v_excentric <N/1
  Sum8/1 -> v_excentric <N/2
  Curvature1/1 -> Sum8/2
  Constant4/1 -> Sum8/1, Sum7/2
  1/1 -> Curvature1/1, Sum7/1
  Sum3/1 -> v_concentric/2
  Sum4/1 -> v_concentric/1
  Constant1/1 -> Sum3/1, Sum4/2
  Curvature/1 -> Sum3/2

== system nms_model/Muscle Actuation Layer/R TA/PE force-length relation ==
  note: Parallel Elasticity PE
  lce [lopt] : Inport  OutDataType=sfix(16)  OutScaling=2^0
  Constant3 : Constant  OutDataType=sfix(16)  OutScaling=2^0
  Math Function2 : Math  Operator=square  OutDataType=sfix(16)  OutScaling=2^0  SaturateOnIntegerOverflow=on
  Mux : Mux  Inputs=2
  Sum1 : Sum  Inputs=|+-  OutDataType=sfix(16)  OutScaling=2^0  SaturateOnIntegerOverflow=on  InputSameDT=on  OutDataTypeStr=Inherit: Same as first input
  force above slack length : Fcn  Expr=u(2) * (u(1)>1)
  reference strain [lopt] : Constant  Value=w  OutDataType=sfix(16)  OutScaling=2^0
  relative strain : Product  Inputs=*/  OutDataType=sfix(16)  OutScaling=2^-10
  fpe [Fmax] : Outport  OutDataType=sfix(16)  OutScaling=2^0
  wires:
  Mux/1 -> force above slack length/1
  lce [lopt]/1 -> Mux/1, Sum1/1
  Constant3/1 -> Sum1/2
  Sum1/1 -> relative strain/1
  reference strain [lopt]/1 -> relative strain/2
  relative strain/1 -> Math Function2/1
  Math Function2/1 -> Mux/2
  force above slack length/1 -> fpe [Fmax]/1

== system nms_model/Muscle Actuation Layer/R TA/SE force-length relation ==
  note: SE Force-Length Relationship
  lse [lslack] : Inport  OutDataType=sfix(16)  OutScaling=2^0
  Constant1 : Constant  OutDataType=sfix(16)  OutScaling=2^0
  Math Function : Math  Operator=square  OutDataType=sfix(16)  OutScaling=2^0  SaturateOnIntegerOverflow=on
  Mux : Mux  Inputs=2
  Sum4 : Sum  Inputs=|+-  OutDataType=sfix(16)  OutScaling=2^0  SaturateOnIntegerOverflow=on  InputSameDT=on  OutDataTypeStr=Inherit: Same as first input
  force above slack length : Fcn  Expr=u(2)*(u(1)>1)
  reference strain [lslack] : Constant  Value=eref  OutDataType=sfix(16)  OutScaling=2^0
  relative strain : Product  Inputs=*/  OutDataType=sfix(16)  OutScaling=2^-10
  fse [Fmax] : Outport  OutDataType=sfix(16)  OutScaling=2^0
  wires:
  Mux/1 -> force above slack length/1
  force above slack length/1 -> fse [Fmax]/1
  Math Function/1 -> Mux/2
  lse [lslack]/1 -> Mux/1, Sum4/1
  relative strain/1 -> Math Function/1
  reference strain [lslack]/1 -> relative strain/2
  Sum4/1 -> relative strain/1
  Constant1/1 -> Sum4/2

== system nms_model/Muscle Actuation Layer/R VAS/BE force-length relation ==
  note: Buffer Elasticity BE
  lce [lopt] : Inport  OutDataType=sfix(16)  OutScaling=2^0
  Constant1 : Constant  Value=1-w  OutDataType=sfix(16)  OutScaling=2^0
  Math Function : Math  Operator=square  OutDataType=sfix(16)  OutScaling=2^0  SaturateOnIntegerOverflow=on
  Mux1 : Mux  Inputs=2
  Sum4 : Sum  Inputs=|+-  OutDataType=sfix(16)  OutScaling=2^0  SaturateOnIntegerOverflow=on  InputSameDT=on  OutDataTypeStr=Inherit: Same as first input
  force above slack length : Fcn  Expr=u(2)*(u(1)<0)
  reference strain [lslack] : Constant  Value=w/2  OutDataType=sfix(16)  OutScaling=2^0
  relative strain : Product  Inputs=*/  OutDataType=sfix(16)  OutScaling=2^-10
  fbe [Fmax] : Outport  OutDataType=sfix(16)  OutScaling=2^0
  wires:
  lce [lopt]/1 -> Sum4/1
  Mux1/1 -> force above slack length/1
  force above slack length/1 -> fbe [Fmax]/1
  Math Function/1 -> Mux1/2
  relative strain/1 -> Math Function/1
  reference strain [lslack]/1 -> relative strain/2
  Sum4/1 -> relative strain/1, Mux1/1
  Constant1/1 -> Sum4/2

== system nms_model/Muscle Actuation Layer/R VAS/CE force-length relation ==
  note: CE Force-Length Relationship
  lce [lopt] : Inport  OutDataType=sfix(16)  OutScaling=2^0
  Abs : Abs
  Constant1 : Constant  OutDataType=sfix(16)  OutScaling=2^0
  Constant2 : Constant  Value=3  OutDataType=sfix(16)  OutScaling=2^0
  Gain : Gain  Gain=log(c)  ParameterDataType=sfix(16)  ParameterScaling=2^0  OutDataType=sfix(16)  OutScaling=2^0
  Math Function : Math  OutDataType=sfix(16)  OutScaling=2^0  SaturateOnIntegerOverflow=on
  Math Function1 : Math  Operator=pow  OutDataType=sfix(16)  OutScaling=2^0  SaturateOnIntegerOverflow=on
  Sum4 : Sum  Inputs=|+-  OutDataType=sfix(16)  OutScaling=2^0  SaturateOnIntegerOverflow=on  InputSameDT=on  OutDataTypeStr=Inherit: Same as first input
  normalized position : Product  Inputs=*/  OutDataType=sfix(16)  OutScaling=2^-10
  relative width : Constant  Value=w  OutDataType=sfix(16)  OutScaling=2^0
  fce [Fmax] : Outport  OutDataType=sfix(16)  OutScaling=2^0
  wires:
  lce [lopt]/1 -> Sum4/1
  relative width/1 -> normalized position/2
  Constant1/1 -> Sum4/2
  Sum4/1 -> Abs/1
  Abs/1 -> normalized position/1
  normalized position/1 -> Math Function1/1
  Constant2/1 -> Math Function1/2
  Math Function1/1 -> Gain/1
  Gain/1 -> Math Function/1
  Math Function/1 -> fce [Fmax]/1

== system nms_model/Muscle Actuation Layer/R VAS/CE inverse  force-velocity relation ==
  note: CE Inverse Force-Velocity Relationship
  Fv[Fmax] : Inport  OutDataType=sfix(16)  OutScaling=2^0
  1 : Product  Inputs=/*  OutDataType=sfix(16)  OutScaling=2^-10
  Constant{1,3..4,8} (4 alike) : Constant  OutDataType=sfix(16)  OutScaling=2^0
  Constant2 : Constant  Value=N  OutDataType=sfix(16)  OutScaling=2^0
  Constant5 : Constant  Value=N  OutDataType=sfix(16)  OutScaling=2^0
  Curvature : Gain  Gain=K  ParameterDataType=sfix(16)  ParameterScaling=2^0  OutDataType=sfix(16)  OutScaling=2^0  SaturateOnIntegerOverflow=on  OutDataTypeStr=Inherit: Same as input  ParamDataTypeStr=Inherit: Same as input
  Curvature1 : Gain  Gain=7.56*K  ParameterDataType=sfix(16)  ParameterScaling=2^0  OutDataType=sfix(16)  OutScaling=2^0  SaturateOnIntegerOverflow=on  OutDataTypeStr=Inherit: Same as input  ParamDataTypeStr=Inherit: Same as input
  Mux : Mux  Inputs=2
  Mux1 : Mux  Inputs=3
  Mux2 : Mux  Inputs=3
  Slope : Gain  Gain=1e-2  ParameterDataType=sfix(16)  ParameterScaling=2^0  OutDataType=sfix(16)  OutScaling=2^0  SaturateOnIntegerOverflow=on  OutDataTypeStr=Inherit: Same as input  ParamDataTypeStr=Inherit: Same as input
  Sum1 : Sum  Inputs=|++  OutDataType=sfix(16)  OutScaling=2^0  SaturateOnIntegerOverflow=on  InputSameDT=on  OutDataTypeStr=Inherit: Same as first input
  Sum2 : Sum  OutDataType=sfix(16)  OutScaling=2^0  SaturateOnIntegerOverflow=on  InputSameDT=on  OutDataTypeStr=Inherit: Same as first input
  Sum3 : Sum  Inputs=++|  OutDataType=sfix(16)  OutScaling=2^0  SaturateOnIntegerOverflow=on  InputSameDT=on  OutDataTypeStr=Inherit: Same as first input
  Sum4 : Sum  Inputs=|+-  OutDataType=sfix(16)  OutScaling=2^0  SaturateOnIntegerOverflow=on  InputSameDT=on  OutDataTypeStr=Inherit: Same as first input
  Sum5 : Sum  Inputs=|-+  OutDataType=sfix(16)  OutScaling=2^0  SaturateOnIntegerOverflow=on  InputSameDT=on  OutDataTypeStr=Inherit: Same as first input
  Sum6 : Sum  Inputs=-+|  OutDataType=sfix(16)  OutScaling=2^0  SaturateOnIntegerOverflow=on  InputSameDT=on  OutDataTypeStr=Inherit: Same as first input
  Sum7 : Sum  Inputs=|++  OutDataType=sfix(16)  OutScaling=2^0  SaturateOnIntegerOverflow=on  InputSameDT=on  OutDataTypeStr=Inherit: Same as first input
  Sum8 : Sum  Inputs=+-|  OutDataType=sfix(16)  OutScaling=2^0  SaturateOnIntegerOverflow=on  InputSameDT=on  OutDataTypeStr=Inherit: Same as first input
  Sum9 : Sum  OutDataType=sfix(16)  OutScaling=2^0  SaturateOnIntegerOverflow=on  InputSameDT=on  OutDataTypeStr=Inherit: Same as first input
  concentric branch : Fcn  Expr=u(1) * (u(2)<=1)
  excentric branch : Fcn  Expr=u(2) * (u(1)>1)*(u(1)<=u(3))
  excentric overshoot : Fcn  Expr=u(3) * (u(2)>u(1))
  v_concentric : Product  Inputs=*/  OutDataType=sfix(16)  OutScaling=2^-10
  v_excentric <N : Product  Inputs=*/  OutDataType=sfix(16)  OutScaling=2^-10
  v[vmax] : Outport  OutDataType=sfix(16)  OutScaling=2^0
  wires:
  Curvature/1 -> Sum3/2
  Constant1/1 -> Sum4/2, Sum3/1
  Sum4/1 -> v_concentric/1
  Sum3/1 -> v_concentric/2
  1/1 -> Sum7/1, Curvature1/1
  Constant4/1 -> Sum7/2, Sum8/1
  Curvature1/1 -> Sum8/2
  Sum8/1 -> v_excentric <N/2
  Sum7/1 -> v_excentric <N/1
  v_concentric/1 -> Mux/1
  Fv[Fmax]/1 -> Sum4/1, Curvature/1, Sum6/2, Mux/2, Mux1/1, Mux2/2
  Sum9/1 -> v[vmax]/1
  Sum2/1 -> Sum9/2
  excentric overshoot/1 -> Sum2/2
  Slope/1 -> Sum1/1
  Constant8/1 -> Sum1/2
  Sum6/1 -> 1/2, Slope/1
  Constant2/1 -> Sum6/1, Sum5/2
  Sum5/1 -> 1/1
  Constant3/1 -> Sum5/1
  Mux/1 -> concentric branch/1
  Mux1/1 -> excentric branch/1
  v_excentric <N/1 -> Mux1/2
  Mux2/1 -> excentric overshoot/1
  concentric branch/1 -> Sum9/1
  excentric branch/1 -> Sum2/1
  Constant5/1 -> Mux1/3, Mux2/1
  Sum1/1 -> Mux2/3

== system nms_model/Muscle Actuation Layer/R VAS/PE force-length relation ==
  note: Parallel Elasticity PE
  lce [lopt] : Inport  OutDataType=sfix(16)  OutScaling=2^0
  Constant3 : Constant  OutDataType=sfix(16)  OutScaling=2^0
  Math Function2 : Math  Operator=square  OutDataType=sfix(16)  OutScaling=2^0  SaturateOnIntegerOverflow=on
  Mux : Mux  Inputs=2
  Sum1 : Sum  Inputs=|+-  OutDataType=sfix(16)  OutScaling=2^0  SaturateOnIntegerOverflow=on  InputSameDT=on  OutDataTypeStr=Inherit: Same as first input
  force above slack length : Fcn  Expr=u(2) * (u(1)>1)
  reference strain [lopt] : Constant  Value=w  OutDataType=sfix(16)  OutScaling=2^0
  relative strain : Product  Inputs=*/  OutDataType=sfix(16)  OutScaling=2^-10
  fpe [Fmax] : Outport  OutDataType=sfix(16)  OutScaling=2^0
  wires:
  Mux/1 -> force above slack length/1
  lce [lopt]/1 -> Mux/1, Sum1/1
  Constant3/1 -> Sum1/2
  Sum1/1 -> relative strain/1
  reference strain [lopt]/1 -> relative strain/2
  relative strain/1 -> Math Function2/1
  Math Function2/1 -> Mux/2
  force above slack length/1 -> fpe [Fmax]/1

== system nms_model/Muscle Actuation Layer/R VAS/SE force-length relation ==
  note: SE Force-Length Relationship
  lse [lslack] : Inport  OutDataType=sfix(16)  OutScaling=2^0
  Constant1 : Constant  OutDataType=sfix(16)  OutScaling=2^0
  Math Function : Math  Operator=square  OutDataType=sfix(16)  OutScaling=2^0  SaturateOnIntegerOverflow=on
  Mux : Mux  Inputs=2
  Sum4 : Sum  Inputs=|+-  OutDataType=sfix(16)  OutScaling=2^0  SaturateOnIntegerOverflow=on  InputSameDT=on  OutDataTypeStr=Inherit: Same as first input
  force above slack length : Fcn  Expr=u(2)*(u(1)>1)
  reference strain [lslack] : Constant  Value=eref  OutDataType=sfix(16)  OutScaling=2^0
  relative strain : Product  Inputs=*/  OutDataType=sfix(16)  OutScaling=2^-10
  fse [Fmax] : Outport  OutDataType=sfix(16)  OutScaling=2^0
  wires:
  Mux/1 -> force above slack length/1
  force above slack length/1 -> fse [Fmax]/1
  Math Function/1 -> Mux/2
  lse [lslack]/1 -> Mux/1, Sum4/1
  relative strain/1 -> Math Function/1
  reference strain [lslack]/1 -> relative strain/2
  Sum4/1 -> relative strain/1
  Constant1/1 -> Sum4/2

== system nms_model/Body Mechanics Layer/Left Ball Contact/Ground Friction Model/Friction Switch ==
  note: Static/Kinetic Friction Switch
  Slide! : Inport  OutDataType=sfix(16)  OutScaling=2^0
  Stick! : Inport  Port=2  OutDataType=sfix(16)  OutScaling=2^0
  Memory : Memory
  S-R Flip-Flop : simulink_extras/Flip Flops/S-R Flip-Flop  SystemSampleTime=-1  initial_condition=1
  Terminator : Terminator
  Stiction : Outport  OutDataType=sfix(16)  OutScaling=2^0
  wires:
  S-R Flip-Flop/1 -> Memory/1
  S-R Flip-Flop/2 -> Terminator/1
  Stick!/1 -> S-R Flip-Flop/1
  Slide!/1 -> S-R Flip-Flop/2
  Memory/1 -> Stiction/1
